simulink model "thirdscheme"  (R2022a)
settings: Solver=VariableStepAuto  StartTime=0.0  StopTime=12.0  RelTol=1e-3
libraries: commsequence2 x1, commseqgen3 x1, commutil2 x1
settings Model: Creator=Admin  LastModifiedBy=Admin

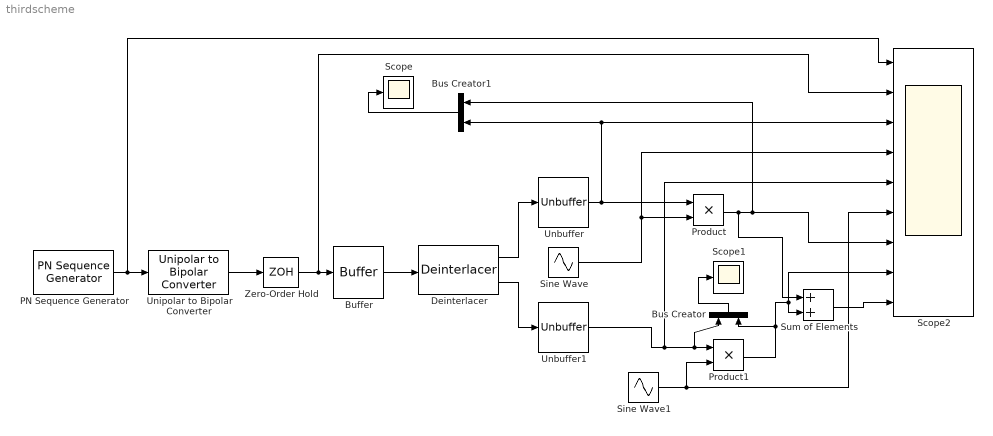
== system thirdscheme ==
  Buffer : Buffer  N=2  OutputFrames=off
  Bus Creator : BusCreator  Inputs=2
  Bus Creator1 : BusCreator  Inputs=2
  Deinterlacer : commsequence2/Deinterlacer
      settings: SourceProductBaseCode=CM
  PN Sequence Generator : commseqgen3/PN Sequence Generator  poly='z^6 + z + 1'  ini_sta=[0 0 0 0 0 1]  outBitMaskSource=Input port  shift=0  outVarSiz=off  maxOutSizeMode=Dialog parameter  maxOutSize=[10 1]  Ts=1/1200  sampPerFrame=1  reset=off  bitPackedOutputs=off  outDataType=double  numPackedBits=8  bitPackDataSigned=off  bitPackedOutDType=double
  Product : Product
  Product1 : Product
  Scope : Scope
  Scope1 : Scope
  Scope2 : Scope  NumInputPorts=9
  Sine Wave : Sin  Frequency=753600  Phase=pi/2  SampleTime=0
  Sine Wave1 : Sin  Frequency=753600  SampleTime=0
  Sum of Elements : Sum
  Unbuffer : Unbuffer
  Unbuffer1 : Unbuffer
  Unipolar to Bipolar Converter : commutil2/Unipolar to Bipolar Converter  M=2  polarity=Positive  dataType=Inherit via internal rule
  Zero-Order Hold : ZeroOrderHold  SampleTime=-1
  wires:
  PN Sequence Generator/1 -> Scope2/1, Unipolar to Bipolar Converter/1
  Unipolar to Bipolar Converter/1 -> Zero-Order Hold/1
  Zero-Order Hold/1 -> Scope2/2, Buffer/1
  Buffer/1 -> Deinterlacer/1
  Deinterlacer/1 -> Unbuffer/1
  Deinterlacer/2 -> Unbuffer1/1
  Sine Wave1/1 -> Scope2/6, Product1/2
  Unbuffer1/1 -> Scope2/5, Bus Creator/1, Product1/1
  Bus Creator/1 -> Scope1/1
  Product1/1 -> Bus Creator/2, Scope2/8, Sum of Elements/2
  Sum of Elements/1 -> Scope2/9
  Sine Wave/1 -> Scope2/4, Product/2
  Bus Creator1/1 -> Scope/1
  Unbuffer/1 -> Bus Creator1/2, Scope2/3, Product/1
  Product/1 -> Sum of Elements/1, Bus Creator1/1, Scope2/7
